simulink model "average_filter_test"  (R2023b)
settings: Solver=VariableStepAuto  StartTime=0.0  StopTime=10.0  RelTol=1e-3
settings Model: Creator=lxj  LastModifiedBy=lxj

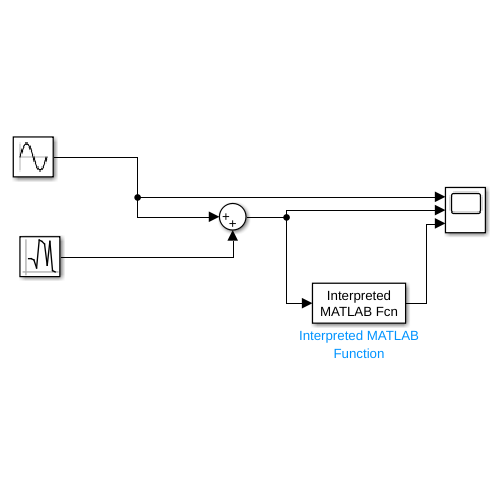
[thumbnail: Simulink's stored preview of the top-level diagram]
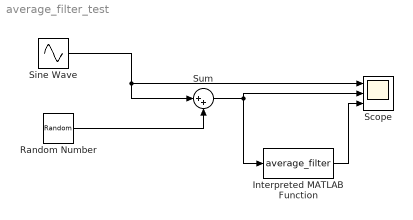
== system average_filter_test ==
  Interpreted MATLAB Function : MATLABFcn  MATLABFcn=average_filter
  Random Number : RandomNumber  Variance=0.01  SampleTime=0.1
  Scope : Scope  NumInputPorts=3
  Sine Wave : Sin  SampleTime=0
  Sum : Sum  Inputs=|++
  wires:
  Random Number/1 -> Sum/2
  Sum/1 -> Interpreted MATLAB Function/1, Scope/2
  Sine Wave/1 -> Scope/1, Sum/1
  Interpreted MATLAB Function/1 -> Scope/3
